simulink model "Simulation_TF_of_Motor"  (R2024b)
settings: Solver=VariableStepAuto  StartTime=0  StopTime=11  RelTol=1e-3
values from neighbouring files (symbols this model uses):
  fc = 40    [SampleCodeCSD_CRP.m]    (also in data for tf of motor 2.mat; data for tf of motor 3.mat; data for tf of motor.mat)
  Ts = 1/fs    (= 0.0125)    [SampleCodeCSD_CRP.m]    (also in data for tf of motor 2.mat; data for tf of motor 3.mat; data for tf of motor.mat)
settings Model: Creator=DONGMO ZEWO  LastModifiedBy=DONGMO ZEWO

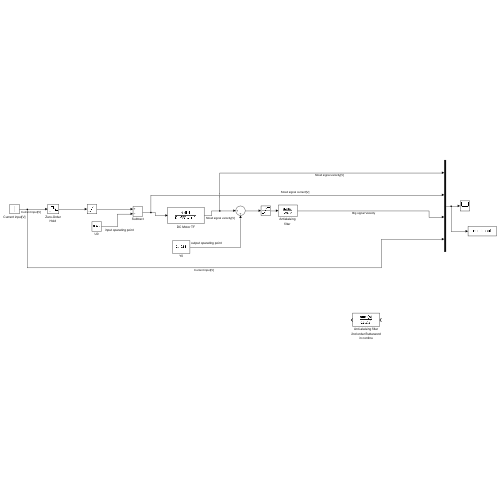
[thumbnail: Simulink's stored preview of the top-level diagram]
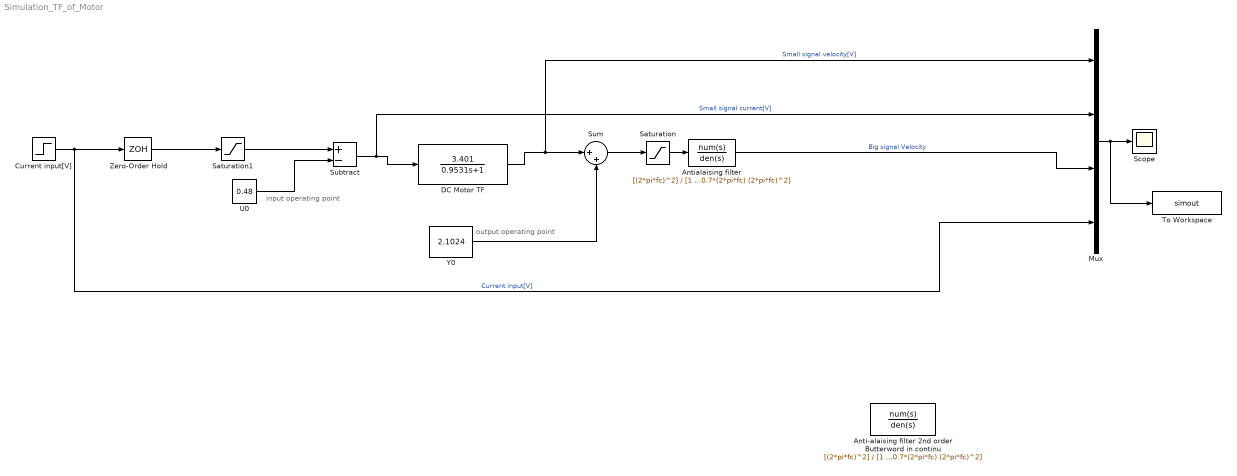
== system Simulation_TF_of_Motor ==
  note: input operating point
  note: output operating point
  Anti-alaising filter 2nd order Butterword in continu : TransferFcn  Numerator=[(2*pi*fc)^2]  Denominator=[1 2*0.7*(2*pi*fc) (2*pi*fc)^2]
  "Antialaising filter " : TransferFcn  Numerator=[(2*pi*fc)^2]  Denominator=[1 2*0.7*(2*pi*fc) (2*pi*fc)^2]
  Current input[V] : Step  Before=0.48  After=0.8  SampleTime=0
  DC Motor TF : TransferFcn  Numerator=[3.401]  Denominator=[0.9531 1]
  Mux : Mux
  Saturation : Saturate  UpperLimit=9  LowerLimit=-9
  Saturation1 : Saturate  UpperLimit=10  LowerLimit=-10
  Scope : Scope
  Subtract : Sum  Inputs=+-
  Sum : Sum  Inputs=|++
  To Workspace : ToWorkspace  VariableName=simout  SaveFormat=Timeseries  SampleTime=-1
  U0 : Constant  Value=0.48  SampleTime=Ts
  Y0 : Constant  Value=2.1024  SampleTime=Ts
  "Zero-Order Hold " : ZeroOrderHold  SampleTime=Ts
  wires:
  DC Motor TF/1 -> Mux/1, Sum/1  "Small signal velocity[V]"
  "Zero-Order Hold "/1 -> Saturation1/1
  Saturation1/1 -> Subtract/1
  U0/1 -> Subtract/2
  Subtract/1 -> Mux/2, DC Motor TF/1  "Small signal current[V]"
  Y0/1 -> Sum/2
  Sum/1 -> Saturation/1
  Saturation/1 -> "Antialaising filter "/1
  Mux/1 -> To Workspace/1, Scope/1
  Current input[V]/1 -> Mux/4, "Zero-Order Hold "/1  "Current input[V]"
  "Antialaising filter "/1 -> Mux/3  "Big signal Velocity"
